simulink model "hx_model_alsop_PID"  (R2017b)
settings: Solver=FixedStepAuto  StartTime=0.0  StopTime=Tsim  FixedStep=ST  RelTol=1e-3
values from neighbouring files (symbols this model uses):
  a1 = N_stages/(3600*Mc)    (= 0.000138888888889)    [main_open_loop_step_responses.m]    (also in main_pida_vs_pid_Fp_dist.m; main_pida_vs_pid_Tci_dist.m; main_pida_vs_pid_Tpi_dist.m; main_pida_vs_pid_sp.m)
  a2 = (U*A)/(3600*Mc*Cpc)    (= 0.010660331384)    [main_open_loop_step_responses.m]    (also in main_pida_vs_pid_Fp_dist.m; main_pida_vs_pid_Tci_dist.m; main_pida_vs_pid_Tpi_dist.m; main_pida_vs_pid_sp.m)
  a3 = N_stages/(3600*Mp)    (= 0.00037037037037)    [main_open_loop_step_responses.m]    (also in main_pida_vs_pid_Fp_dist.m; main_pida_vs_pid_Tci_dist.m; main_pida_vs_pid_Tpi_dist.m; main_pida_vs_pid_sp.m)
  a4 = (U*A)/(3600*Mp*Cpp)    (= 0.0341130604288)    [main_open_loop_step_responses.m]    (also in main_pida_vs_pid_Fp_dist.m; main_pida_vs_pid_Tci_dist.m; main_pida_vs_pid_Tpi_dist.m; main_pida_vs_pid_sp.m)
  Fc = 2500/7936.64    (= 0.314994758487)    [main_open_loop_step_responses.m]    (also in main_pida_vs_pid_Fp_dist.m; main_pida_vs_pid_Tci_dist.m; main_pida_vs_pid_Tpi_dist.m; main_pida_vs_pid_sp.m)
  Fc_min = 500/7936.64    (= 0.0629989516974)    [main_open_loop_step_responses.m]    (also in main_pida_vs_pid_Fp_dist.m; main_pida_vs_pid_Tci_dist.m; main_pida_vs_pid_Tpi_dist.m; main_pida_vs_pid_sp.m)
  Fp = 1500/7936.64    (= 0.188996855092)    [main_open_loop_step_responses.m]    (also in main_pida_vs_pid_Fp_dist.m; main_pida_vs_pid_Tci_dist.m; main_pida_vs_pid_Tpi_dist.m; main_pida_vs_pid_sp.m)
  Kp = KpPID    [main_pida_vs_pid_Fp_dist.m]    (also in main_pida_vs_pid_Tci_dist.m; main_pida_vs_pid_Tpi_dist.m; main_pida_vs_pid_sp.m)
  N = 10    [main_pida_vs_pid_Fp_dist.m]    (also in main_pida_vs_pid_Tci_dist.m; main_pida_vs_pid_Tpi_dist.m; main_pida_vs_pid_sp.m; main_tuning_pid.m = 20)
  noise_max = 0.5    [main_pida_vs_pid_Fp_dist.m]    (also in main_pida_vs_pid_Tci_dist.m; main_pida_vs_pid_Tpi_dist.m; main_pida_vs_pid_sp.m)
  noise_min = -0.5    [main_pida_vs_pid_Fp_dist.m]    (also in main_pida_vs_pid_Tci_dist.m; main_pida_vs_pid_Tpi_dist.m; main_pida_vs_pid_sp.m)
  step_Fp = 0    [main_open_loop_step_responses.m]    (also in main_pida_vs_pid_Fp_dist.m = 0.0125; main_pida_vs_pid_Tci_dist.m; main_pida_vs_pid_Tpi_dist.m; main_pida_vs_pid_sp.m)
  step_Tci = 0    [main_open_loop_step_responses.m]    (also in main_pida_vs_pid_Fp_dist.m; main_pida_vs_pid_Tci_dist.m = 2.5; main_pida_vs_pid_Tpi_dist.m; main_pida_vs_pid_sp.m)
  step_time = 0    [main_open_loop_step_responses.m]    (also in main_pida_vs_pid_Fp_dist.m; main_pida_vs_pid_Tci_dist.m; main_pida_vs_pid_Tpi_dist.m; main_pida_vs_pid_sp.m)
  step_Tpi = 0    [main_open_loop_step_responses.m]    (also in main_pida_vs_pid_Fp_dist.m; main_pida_vs_pid_Tci_dist.m; main_pida_vs_pid_Tpi_dist.m = 2.5; main_pida_vs_pid_sp.m)
  step_Tpo = 0    [main_open_loop_step_responses.m]    (also in main_pida_vs_pid_Fp_dist.m; main_pida_vs_pid_Tci_dist.m; main_pida_vs_pid_Tpi_dist.m; main_pida_vs_pid_sp.m = -2.5)
  Tci = 294.26    [main_open_loop_step_responses.m]    (also in main_pida_vs_pid_Fp_dist.m; main_pida_vs_pid_Tci_dist.m; main_pida_vs_pid_Tpi_dist.m; main_pida_vs_pid_sp.m)
  Tco_init1 = Tco_init1.Data(end)    [main_open_loop_step_responses.m]    (also in main_pida_vs_pid_Fp_dist.m; main_pida_vs_pid_Tci_dist.m; main_pida_vs_pid_Tpi_dist.m; main_pida_vs_pid_sp.m)
  Tco_init10 = Tco_init10.Data(end)    [main_open_loop_step_responses.m]    (also in main_pida_vs_pid_Fp_dist.m; main_pida_vs_pid_Tci_dist.m; main_pida_vs_pid_Tpi_dist.m; main_pida_vs_pid_sp.m)
  Tco_init11 = Tco_init11.Data(end)    [main_open_loop_step_responses.m]    (also in main_pida_vs_pid_Fp_dist.m; main_pida_vs_pid_Tci_dist.m; main_pida_vs_pid_Tpi_dist.m; main_pida_vs_pid_sp.m)
  Tco_init12 = Tco_init12.Data(end)    [main_open_loop_step_responses.m]    (also in main_pida_vs_pid_Fp_dist.m; main_pida_vs_pid_Tci_dist.m; main_pida_vs_pid_Tpi_dist.m; main_pida_vs_pid_sp.m)
  Tco_init13 = Tco_init13.Data(end)    [main_open_loop_step_responses.m]    (also in main_pida_vs_pid_Fp_dist.m; main_pida_vs_pid_Tci_dist.m; main_pida_vs_pid_Tpi_dist.m; main_pida_vs_pid_sp.m)
  Tco_init14 = Tco_init14.Data(end)    [main_open_loop_step_responses.m]    (also in main_pida_vs_pid_Fp_dist.m; main_pida_vs_pid_Tci_dist.m; main_pida_vs_pid_Tpi_dist.m; main_pida_vs_pid_sp.m)
  Tco_init15 = Tco_init15.Data(end)    [main_open_loop_step_responses.m]    (also in main_pida_vs_pid_Fp_dist.m; main_pida_vs_pid_Tci_dist.m; main_pida_vs_pid_Tpi_dist.m; main_pida_vs_pid_sp.m)
  Tco_init16 = Tco_init16.Data(end)    [main_open_loop_step_responses.m]    (also in main_pida_vs_pid_Fp_dist.m; main_pida_vs_pid_Tci_dist.m; main_pida_vs_pid_Tpi_dist.m; main_pida_vs_pid_sp.m)
  Tco_init17 = Tco_init17.Data(end)    [main_open_loop_step_responses.m]    (also in main_pida_vs_pid_Fp_dist.m; main_pida_vs_pid_Tci_dist.m; main_pida_vs_pid_Tpi_dist.m; main_pida_vs_pid_sp.m)
  Tco_init18 = Tco_init18.Data(end)    [main_open_loop_step_responses.m]    (also in main_pida_vs_pid_Fp_dist.m; main_pida_vs_pid_Tci_dist.m; main_pida_vs_pid_Tpi_dist.m; main_pida_vs_pid_sp.m)
  Tco_init19 = Tco_init19.Data(end)    [main_open_loop_step_responses.m]    (also in main_pida_vs_pid_Fp_dist.m; main_pida_vs_pid_Tci_dist.m; main_pida_vs_pid_Tpi_dist.m; main_pida_vs_pid_sp.m)
  Tco_init2 = Tco_init2.Data(end)    [main_open_loop_step_responses.m]    (also in main_pida_vs_pid_Fp_dist.m; main_pida_vs_pid_Tci_dist.m; main_pida_vs_pid_Tpi_dist.m; main_pida_vs_pid_sp.m)
  Tco_init20 = Tco_init20.Data(end)    [main_open_loop_step_responses.m]    (also in main_pida_vs_pid_Fp_dist.m; main_pida_vs_pid_Tci_dist.m; main_pida_vs_pid_Tpi_dist.m; main_pida_vs_pid_sp.m)
  Tco_init3 = Tco_init3.Data(end)    [main_open_loop_step_responses.m]    (also in main_pida_vs_pid_Fp_dist.m; main_pida_vs_pid_Tci_dist.m; main_pida_vs_pid_Tpi_dist.m; main_pida_vs_pid_sp.m)
  Tco_init4 = Tco_init4.Data(end)    [main_open_loop_step_responses.m]    (also in main_pida_vs_pid_Fp_dist.m; main_pida_vs_pid_Tci_dist.m; main_pida_vs_pid_Tpi_dist.m; main_pida_vs_pid_sp.m)
  Tco_init5 = Tco_init5.Data(end)    [main_open_loop_step_responses.m]    (also in main_pida_vs_pid_Fp_dist.m; main_pida_vs_pid_Tci_dist.m; main_pida_vs_pid_Tpi_dist.m; main_pida_vs_pid_sp.m)
  Tco_init6 = Tco_init6.Data(end)    [main_open_loop_step_responses.m]    (also in main_pida_vs_pid_Fp_dist.m; main_pida_vs_pid_Tci_dist.m; main_pida_vs_pid_Tpi_dist.m; main_pida_vs_pid_sp.m)
  Tco_init7 = Tco_init7.Data(end)    [main_open_loop_step_responses.m]    (also in main_pida_vs_pid_Fp_dist.m; main_pida_vs_pid_Tci_dist.m; main_pida_vs_pid_Tpi_dist.m; main_pida_vs_pid_sp.m)
  Tco_init8 = Tco_init8.Data(end)    [main_open_loop_step_responses.m]    (also in main_pida_vs_pid_Fp_dist.m; main_pida_vs_pid_Tci_dist.m; main_pida_vs_pid_Tpi_dist.m; main_pida_vs_pid_sp.m)
  Tco_init9 = Tco_init9.Data(end)    [main_open_loop_step_responses.m]    (also in main_pida_vs_pid_Fp_dist.m; main_pida_vs_pid_Tci_dist.m; main_pida_vs_pid_Tpi_dist.m; main_pida_vs_pid_sp.m)
  Td = TdPID    [main_pida_vs_pid_Fp_dist.m]    (also in main_pida_vs_pid_Tci_dist.m; main_pida_vs_pid_Tpi_dist.m; main_pida_vs_pid_sp.m)
  Ti = TiPID    [main_pida_vs_pid_Fp_dist.m]    (also in main_pida_vs_pid_Tci_dist.m; main_pida_vs_pid_Tpi_dist.m; main_pida_vs_pid_sp.m)
  Tpi = 366.48    [main_open_loop_step_responses.m]    (also in main_pida_vs_pid_Fp_dist.m; main_pida_vs_pid_Tci_dist.m; main_pida_vs_pid_Tpi_dist.m; main_pida_vs_pid_sp.m)
  Tpo_init = (Tpo_init1 - 32)*(5/9) + 273.15    [main_open_loop_step_responses.m]    (also in main_pida_vs_pid_Fp_dist.m; main_pida_vs_pid_Tci_dist.m; main_pida_vs_pid_Tpi_dist.m; main_pida_vs_pid_sp.m)
  Tpo_init1 = Tpo_init1.Data(end)    [main_open_loop_step_responses.m]    (also in main_pida_vs_pid_Fp_dist.m; main_pida_vs_pid_Tci_dist.m; main_pida_vs_pid_Tpi_dist.m; main_pida_vs_pid_sp.m)
  Tpo_init10 = Tpo_init10.Data(end)    [main_open_loop_step_responses.m]    (also in main_pida_vs_pid_Fp_dist.m; main_pida_vs_pid_Tci_dist.m; main_pida_vs_pid_Tpi_dist.m; main_pida_vs_pid_sp.m)
  Tpo_init11 = Tpo_init11.Data(end)    [main_open_loop_step_responses.m]    (also in main_pida_vs_pid_Fp_dist.m; main_pida_vs_pid_Tci_dist.m; main_pida_vs_pid_Tpi_dist.m; main_pida_vs_pid_sp.m)
  Tpo_init12 = Tpo_init12.Data(end)    [main_open_loop_step_responses.m]    (also in main_pida_vs_pid_Fp_dist.m; main_pida_vs_pid_Tci_dist.m; main_pida_vs_pid_Tpi_dist.m; main_pida_vs_pid_sp.m)
  Tpo_init13 = Tpo_init13.Data(end)    [main_open_loop_step_responses.m]    (also in main_pida_vs_pid_Fp_dist.m; main_pida_vs_pid_Tci_dist.m; main_pida_vs_pid_Tpi_dist.m; main_pida_vs_pid_sp.m)
  Tpo_init14 = Tpo_init14.Data(end)    [main_open_loop_step_responses.m]    (also in main_pida_vs_pid_Fp_dist.m; main_pida_vs_pid_Tci_dist.m; main_pida_vs_pid_Tpi_dist.m; main_pida_vs_pid_sp.m)
  Tpo_init15 = Tpo_init15.Data(end)    [main_open_loop_step_responses.m]    (also in main_pida_vs_pid_Fp_dist.m; main_pida_vs_pid_Tci_dist.m; main_pida_vs_pid_Tpi_dist.m; main_pida_vs_pid_sp.m)
  Tpo_init16 = Tpo_init16.Data(end)    [main_open_loop_step_responses.m]    (also in main_pida_vs_pid_Fp_dist.m; main_pida_vs_pid_Tci_dist.m; main_pida_vs_pid_Tpi_dist.m; main_pida_vs_pid_sp.m)
  Tpo_init17 = Tpo_init17.Data(end)    [main_open_loop_step_responses.m]    (also in main_pida_vs_pid_Fp_dist.m; main_pida_vs_pid_Tci_dist.m; main_pida_vs_pid_Tpi_dist.m; main_pida_vs_pid_sp.m)
  Tpo_init18 = Tpo_init18.Data(end)    [main_open_loop_step_responses.m]    (also in main_pida_vs_pid_Fp_dist.m; main_pida_vs_pid_Tci_dist.m; main_pida_vs_pid_Tpi_dist.m; main_pida_vs_pid_sp.m)
  Tpo_init19 = Tpo_init19.Data(end)    [main_open_loop_step_responses.m]    (also in main_pida_vs_pid_Fp_dist.m; main_pida_vs_pid_Tci_dist.m; main_pida_vs_pid_Tpi_dist.m; main_pida_vs_pid_sp.m)
  Tpo_init2 = Tpo_init2.Data(end)    [main_open_loop_step_responses.m]    (also in main_pida_vs_pid_Fp_dist.m; main_pida_vs_pid_Tci_dist.m; main_pida_vs_pid_Tpi_dist.m; main_pida_vs_pid_sp.m)
  Tpo_init20 = Tpo_init20.Data(end)    [main_open_loop_step_responses.m]    (also in main_pida_vs_pid_Fp_dist.m; main_pida_vs_pid_Tci_dist.m; main_pida_vs_pid_Tpi_dist.m; main_pida_vs_pid_sp.m)
  Tpo_init3 = Tpo_init3.Data(end)    [main_open_loop_step_responses.m]    (also in main_pida_vs_pid_Fp_dist.m; main_pida_vs_pid_Tci_dist.m; main_pida_vs_pid_Tpi_dist.m; main_pida_vs_pid_sp.m)
  Tpo_init4 = Tpo_init4.Data(end)    [main_open_loop_step_responses.m]    (also in main_pida_vs_pid_Fp_dist.m; main_pida_vs_pid_Tci_dist.m; main_pida_vs_pid_Tpi_dist.m; main_pida_vs_pid_sp.m)
  Tpo_init5 = Tpo_init5.Data(end)    [main_open_loop_step_responses.m]    (also in main_pida_vs_pid_Fp_dist.m; main_pida_vs_pid_Tci_dist.m; main_pida_vs_pid_Tpi_dist.m; main_pida_vs_pid_sp.m)
  Tpo_init6 = Tpo_init6.Data(end)    [main_open_loop_step_responses.m]    (also in main_pida_vs_pid_Fp_dist.m; main_pida_vs_pid_Tci_dist.m; main_pida_vs_pid_Tpi_dist.m; main_pida_vs_pid_sp.m)
  Tpo_init7 = Tpo_init7.Data(end)    [main_open_loop_step_responses.m]    (also in main_pida_vs_pid_Fp_dist.m; main_pida_vs_pid_Tci_dist.m; main_pida_vs_pid_Tpi_dist.m; main_pida_vs_pid_sp.m)
  Tpo_init8 = Tpo_init8.Data(end)    [main_open_loop_step_responses.m]    (also in main_pida_vs_pid_Fp_dist.m; main_pida_vs_pid_Tci_dist.m; main_pida_vs_pid_Tpi_dist.m; main_pida_vs_pid_sp.m)
  Tpo_init9 = Tpo_init9.Data(end)    [main_open_loop_step_responses.m]    (also in main_pida_vs_pid_Fp_dist.m; main_pida_vs_pid_Tci_dist.m; main_pida_vs_pid_Tpi_dist.m; main_pida_vs_pid_sp.m)
  Wgc = WcpPID    [main_pida_vs_pid_Fp_dist.m]    (also in main_pida_vs_pid_Tci_dist.m; main_pida_vs_pid_Tpi_dist.m; main_pida_vs_pid_sp.m)
  x_eq = -(A_f\(B_f*Fc))    [main_pida_vs_pid_Fp_dist.m]    (also in main_pida_vs_pid_Tci_dist.m; main_pida_vs_pid_Tpi_dist.m; main_pida_vs_pid_sp.m)
undefined symbols (not defined in the file or in its folder): A_f, B_f, C_f, D_f
(part 1 of 2)
settings Model: Creator=Michele  LastModifiedBy=Michele

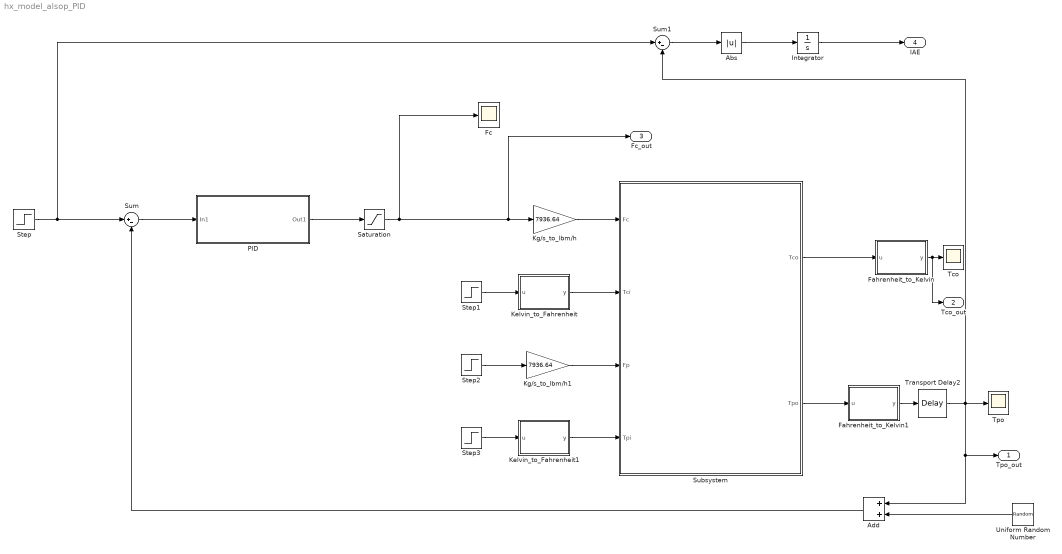
== system hx_model_alsop_PID ==
  Abs : Abs
  Add : Sum
  Fahrenheit_to_Kelvin : MATLAB Function  TreatAsAtomicUnit=on
  Fahrenheit_to_Kelvin1 : MATLAB Function  TreatAsAtomicUnit=on
  Fc : Scope
  Integrator : Integrator
  Kelvin_to_Fahrenheit : MATLAB Function  TreatAsAtomicUnit=on
  Kelvin_to_Fahrenheit1 : MATLAB Function  TreatAsAtomicUnit=on
  Kg/s_to_lbm/h : Gain  Gain=7936.64
  Kg/s_to_lbm/h1 : Gain  Gain=7936.64
  PID : Subsystem
  Saturation : Saturate  UpperLimit=inf  LowerLimit=Fc_min
  Step : Step  Time=step_time  Before=Tpo_init  After=Tpo_init+step_Tpo  SampleTime=0
  Step1 : Step  Time=step_time  Before=Tci  After=Tci+step_Tci  SampleTime=0
  Step2 : Step  Time=step_time  Before=Fp  After=Fp+step_Fp  SampleTime=0
  Step3 : Step  Time=step_time  Before=Tpi  After=Tpi+step_Tpi  SampleTime=0
  Subsystem : Subsystem
  Sum : Sum  Inputs=|+-
  Sum1 : Sum  Inputs=|+-
  Tco : Scope
  Tpo : Scope
  Transport Delay2 : TransportDelay  DelayTime=35  InitialOutput=(Tpo_init1 - 32)*(5/9) + 273.15
  Uniform Random Number : UniformRandomNumber  Minimum=noise_min  Maximum=noise_max  SampleTime=0.1
  Tpo_out : Outport
  Tco_out : Outport  Port=2
  Fc_out : Outport  Port=3
  IAE : Outport  Port=4
  wires:
  Step2/1 -> Kg/s_to_lbm/h1/1
  Step3/1 -> Kelvin_to_Fahrenheit1/1(u)
  Step1/1 -> Kelvin_to_Fahrenheit/1(u)
  Kelvin_to_Fahrenheit/1(y) -> Subsystem/2(Tci)
  Kelvin_to_Fahrenheit1/1(y) -> Subsystem/4(Tpi)
  Fahrenheit_to_Kelvin/1(y) -> Tco_out/1, Tco/1
  Fahrenheit_to_Kelvin1/1(y) -> Transport Delay2/1
  Kg/s_to_lbm/h/1 -> Subsystem/1(Fc)
  Kg/s_to_lbm/h1/1 -> Subsystem/3(Fp)
  Subsystem/1(Tco) -> Fahrenheit_to_Kelvin/1(u)
  Subsystem/2(Tpo) -> Fahrenheit_to_Kelvin1/1(u)
  Saturation/1 -> Fc_out/1, Kg/s_to_lbm/h/1, Fc/1
  PID/1(Out1) -> Saturation/1
  Step/1 -> Sum1/1, Sum/1
  Abs/1 -> Integrator/1
  Sum/1 -> PID/1(In1)
  Integrator/1 -> IAE/1
  Add/1 -> Sum/2
  Uniform Random Number/1 -> Add/2
  Sum1/1 -> Abs/1
  Transport Delay2/1 -> Sum1/2, Tpo/1, Tpo_out/1, Add/1

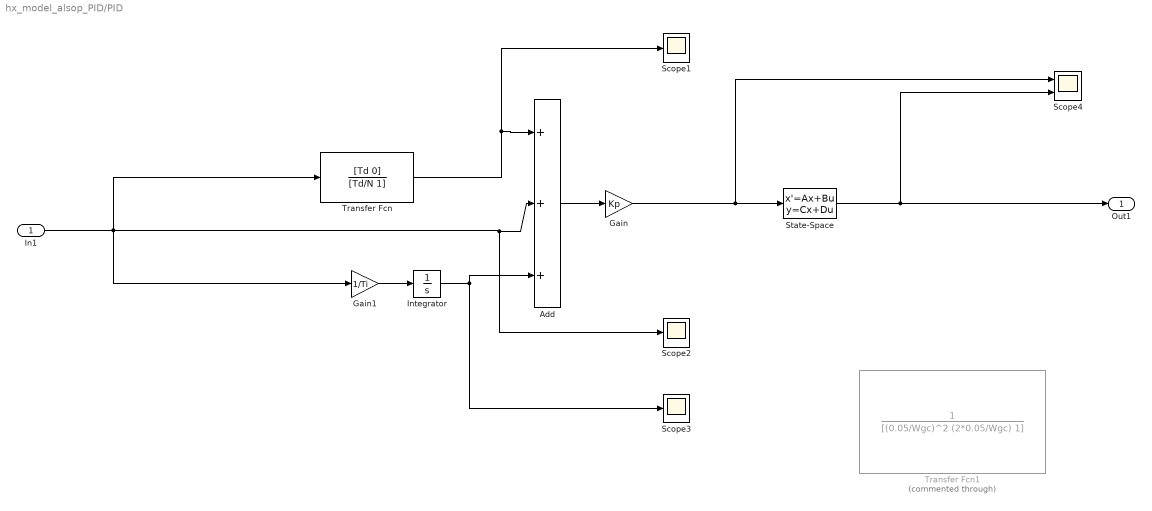
== system hx_model_alsop_PID/PID ==
  In1 : Inport
  Add : Sum  Inputs=+++
  Gain : Gain  Gain=Kp
  Gain1 : Gain  Gain=1/Ti
  Integrator : Integrator  InitialCondition=Fc/Kp
  Scope1 : Scope
  Scope2 : Scope
  Scope3 : Scope
  Scope4 : Scope  NumInputPorts=2
  State-Space : StateSpace  A=A_f  B=B_f  C=C_f  D=D_f  InitialCondition=x_eq
  Transfer Fcn : TransferFcn  Numerator=[Td 0]  Denominator=[Td/N 1]
  Transfer Fcn1 : TransferFcn  Commented=through  Denominator=[(0.05/Wgc)^2 (2*0.05/Wgc) 1]
  Out1 : Outport
  wires:
  Add/1 -> Gain/1
  Integrator/1 -> Add/3, Scope3/1
  Gain1/1 -> Integrator/1
  State-Space/1 -> Scope4/2, Out1/1
  In1/1 -> Transfer Fcn/1, Gain1/1, Add/2, Scope2/1
  Transfer Fcn/1 -> Add/1, Scope1/1
  Gain/1 -> Scope4/1, State-Space/1

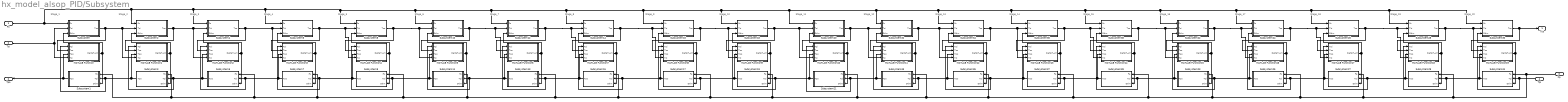
== system hx_model_alsop_PID/Subsystem ==
  note: Stage_1
  note: Stage_2
  note: Stage_3
  note: Stage_4
  note: Stage_5
  note: Stage_6
  note: Stage_7
  note: Stage_8
  note: Stage_9
  note: Stage_10
  note: Stage_13
  note: Stage_20
  note: Stage_16
  note: Stage_11
  note: Stage_18
  note: Stage_15
  note: Stage_19
  note: Stage_12
  note: Stage_17
  note: Stage_14
  Fc : Inport
  Tci : Inport  Port=2
  Fp : Inport  Port=3
  Tpi : Inport  Port=4
  MATLAB Function : MATLAB Function  TreatAsAtomicUnit=on
  MATLAB Function1 : MATLAB Function  TreatAsAtomicUnit=on
  MATLAB Function10 : MATLAB Function  TreatAsAtomicUnit=on
  MATLAB Function11 : MATLAB Function  TreatAsAtomicUnit=on
  MATLAB Function12 : MATLAB Function  TreatAsAtomicUnit=on
  MATLAB Function13 : MATLAB Function  TreatAsAtomicUnit=on
  MATLAB Function14 : MATLAB Function  TreatAsAtomicUnit=on
  MATLAB Function15 : MATLAB Function  TreatAsAtomicUnit=on
  MATLAB Function16 : MATLAB Function  TreatAsAtomicUnit=on
  MATLAB Function17 : MATLAB Function  TreatAsAtomicUnit=on
  MATLAB Function18 : MATLAB Function  TreatAsAtomicUnit=on
  MATLAB Function19 : MATLAB Function  TreatAsAtomicUnit=on
  MATLAB Function2 : MATLAB Function  TreatAsAtomicUnit=on
  MATLAB Function3 : MATLAB Function  TreatAsAtomicUnit=on
  MATLAB Function4 : MATLAB Function  TreatAsAtomicUnit=on
  MATLAB Function5 : MATLAB Function  TreatAsAtomicUnit=on
  MATLAB Function6 : MATLAB Function  TreatAsAtomicUnit=on
  MATLAB Function7 : MATLAB Function  TreatAsAtomicUnit=on
  MATLAB Function8 : MATLAB Function  TreatAsAtomicUnit=on
  MATLAB Function9 : MATLAB Function  TreatAsAtomicUnit=on
  Subsystem : Subsystem
  Subsystem1 : Subsystem
  Subsystem10 : Subsystem
  Subsystem11 : Subsystem
  Subsystem12 : Subsystem
  Subsystem13 : Subsystem
  Subsystem14 : Subsystem
  Subsystem15 : Subsystem
  Subsystem16 : Subsystem
  Subsystem17 : Subsystem
  Subsystem18 : Subsystem
  Subsystem19 : Subsystem
  Subsystem2 : Subsystem
  Subsystem20 : Subsystem
  Subsystem21 : Subsystem
  Subsystem22 : Subsystem
  Subsystem23 : Subsystem
  Subsystem24 : Subsystem
  Subsystem25 : Subsystem
  Subsystem26 : Subsystem
  Subsystem27 : Subsystem
  Subsystem28 : Subsystem
  Subsystem29 : Subsystem
  Subsystem3 : Subsystem
  Subsystem30 : Subsystem
  Subsystem31 : Subsystem
  Subsystem32 : Subsystem
  Subsystem33 : Subsystem
  Subsystem34 : Subsystem
  Subsystem35 : Subsystem
  Subsystem36 : Subsystem
  Subsystem37 : Subsystem
  Subsystem38 : Subsystem
  Subsystem39 : Subsystem
  Subsystem4 : Subsystem
  Subsystem5 : Subsystem
  Subsystem6 : Subsystem
  Subsystem7 : Subsystem
  Subsystem8 : Subsystem
  Subsystem9 : Subsystem
  Tco : Outport
  Tpo : Outport  Port=2
  wires:
  Subsystem1/1(Tpo) -> Tpo/1, MATLAB Function/3(Tpo)
  Subsystem/1(Tco) -> MATLAB Function/2(Tco), MATLAB Function1/4(Tci), Subsystem2/2(Tci)
  MATLAB Function/1(DeltaT_LM) -> Subsystem1/3(Dtlm), Subsystem/3(Dtlm)
  Tci/1 -> MATLAB Function/4(Tci), Subsystem/2(Tci)
  MATLAB Function1/1(DeltaT_LM) -> Subsystem2/3(Dtlm), Subsystem3/3(Dtlm)
  Subsystem2/1(Tco) -> MATLAB Function2/4(Tci), Subsystem4/2(Tci), MATLAB Function1/2(Tco)
  Subsystem3/1(Tpo) -> MATLAB Function/1(Tpi), Subsystem1/2(Tpi), MATLAB Function1/3(Tpo)
  Subsystem4/1(Tco) -> MATLAB Function2/2(Tco), MATLAB Function3/4(Tci), Subsystem6/2(Tci)
  MATLAB Function2/1(DeltaT_LM) -> Subsystem5/3(Dtlm), Subsystem4/3(Dtlm)
  MATLAB Function3/1(DeltaT_LM) -> Subsystem6/3(Dtlm), Subsystem7/3(Dtlm)
  Subsystem6/1(Tco) -> MATLAB Function4/4(Tci), Subsystem8/2(Tci), MATLAB Function3/2(Tco)
  Subsystem8/1(Tco) -> MATLAB Function5/4(Tci), Subsystem10/2(Tci), MATLAB Function4/2(Tco)
  MATLAB Function4/1(DeltaT_LM) -> Subsystem9/3(Dtlm), Subsystem8/3(Dtlm)
  MATLAB Function5/1(DeltaT_LM) -> Subsystem10/3(Dtlm), Subsystem11/3(Dtlm)
  Subsystem10/1(Tco) -> MATLAB Function6/4(Tci), Subsystem12/2(Tci), MATLAB Function5/2(Tco)
  Subsystem12/1(Tco) -> MATLAB Function7/4(Tci), Subsystem14/2(Tci), MATLAB Function6/2(Tco)
  MATLAB Function6/1(DeltaT_LM) -> Subsystem13/3(Dtlm), Subsystem12/3(Dtlm)
  MATLAB Function7/1(DeltaT_LM) -> Subsystem14/3(Dtlm), Subsystem15/3(Dtlm)
  Subsystem14/1(Tco) -> MATLAB Function8/4(Tci), Subsystem16/2(Tci), MATLAB Function7/2(Tco)
  Subsystem16/1(Tco) -> MATLAB Function9/4(Tci), Subsystem18/2(Tci), MATLAB Function8/2(Tco)
  MATLAB Function8/1(DeltaT_LM) -> Subsystem17/3(Dtlm), Subsystem16/3(Dtlm)
  MATLAB Function9/1(DeltaT_LM) -> Subsystem18/3(Dtlm), Subsystem19/3(Dtlm)
  Subsystem5/1(Tpo) -> MATLAB Function2/3(Tpo), MATLAB Function1/1(Tpi), Subsystem3/2(Tpi)
  Subsystem7/1(Tpo) -> MATLAB Function2/1(Tpi), Subsystem5/2(Tpi), MATLAB Function3/3(Tpo)
  Subsystem9/1(Tpo) -> MATLAB Function3/1(Tpi), Subsystem7/2(Tpi), MATLAB Function4/3(Tpo)
  Subsystem11/1(Tpo) -> MATLAB Function4/1(Tpi), Subsystem9/2(Tpi), MATLAB Function5/3(Tpo)
  Subsystem13/1(Tpo) -> MATLAB Function5/1(Tpi), Subsystem11/2(Tpi), MATLAB Function6/3(Tpo)
  Subsystem15/1(Tpo) -> MATLAB Function6/1(Tpi), Subsystem13/2(Tpi), MATLAB Function7/3(Tpo)
  Subsystem17/1(Tpo) -> MATLAB Function7/1(Tpi), Subsystem15/2(Tpi), MATLAB Function8/3(Tpo)
  Subsystem19/1(Tpo) -> MATLAB Function8/1(Tpi), Subsystem17/2(Tpi), MATLAB Function9/3(Tpo)
  Subsystem31/1(Tpo) -> MATLAB Function18/1(Tpi), Subsystem29/2(Tpi), MATLAB Function19/3(Tpo)
  Subsystem32/1(Tco) -> MATLAB Function12/4(Tci), Subsystem34/2(Tci), MATLAB Function11/2(Tco)
  MATLAB Function11/1(DeltaT_LM) -> Subsystem32/3(Dtlm), Subsystem33/3(Dtlm)
  Subsystem25/1(Tpo) -> MATLAB Function15/1(Tpi), Subsystem23/2(Tpi), MATLAB Function16/3(Tpo)
  MATLAB Function15/1(DeltaT_LM) -> Subsystem22/3(Dtlm), Subsystem23/3(Dtlm)
  MATLAB Function12/1(DeltaT_LM) -> Subsystem35/3(Dtlm), Subsystem34/3(Dtlm)
  Subsystem33/1(Tpo) -> MATLAB Function10/1(Tpi), Subsystem21/2(Tpi), MATLAB Function11/3(Tpo)
  MATLAB Function14/1(DeltaT_LM) -> Subsystem39/3(Dtlm), Subsystem38/3(Dtlm)
  Subsystem34/1(Tco) -> MATLAB Function12/2(Tco), MATLAB Function13/4(Tci), Subsystem36/2(Tci)
  Fc/1 -> Subsystem30/1(Fc), Subsystem28/1(Fc), Subsystem26/1(Fc), Subsystem24/1(Fc), Subsystem22/1(Fc), Subsystem38/1(Fc), Subsystem36/1(Fc), Subsystem34/1(Fc), Subsystem32/1(Fc), Subsystem20/1(Fc), Subsystem18/1(Fc), Subsystem16/1(Fc), Subsystem14/1(Fc), Subsystem12/1(Fc), Subsystem10/1(Fc), Subsystem8/1(Fc), Subsystem6/1(Fc), Subsystem4/1(Fc), Subsystem2/1(Fc), Subsystem/1(Fc)
  Subsystem18/1(Tco) -> MATLAB Function9/2(Tco), MATLAB Function10/4(Tci), Subsystem20/2(Tci)
  Subsystem20/1(Tco) -> MATLAB Function10/2(Tco), MATLAB Function11/4(Tci), Subsystem32/2(Tci)
  MATLAB Function10/1(DeltaT_LM) -> Subsystem21/3(Dtlm), Subsystem20/3(Dtlm)
  Subsystem23/1(Tpo) -> MATLAB Function14/1(Tpi), Subsystem39/2(Tpi), MATLAB Function15/3(Tpo)
  Subsystem37/1(Tpo) -> MATLAB Function12/1(Tpi), Subsystem35/2(Tpi), MATLAB Function13/3(Tpo)
  Subsystem38/1(Tco) -> MATLAB Function15/4(Tci), Subsystem22/2(Tci), MATLAB Function14/2(Tco)
  Subsystem21/1(Tpo) -> MATLAB Function10/3(Tpo), MATLAB Function9/1(Tpi), Subsystem19/2(Tpi)
  Subsystem29/1(Tpo) -> MATLAB Function17/1(Tpi), Subsystem27/2(Tpi), MATLAB Function18/3(Tpo)
  Subsystem27/1(Tpo) -> MATLAB Function16/1(Tpi), Subsystem25/2(Tpi), MATLAB Function17/3(Tpo)
  Subsystem22/1(Tco) -> MATLAB Function16/4(Tci), Subsystem24/2(Tci), MATLAB Function15/2(Tco)
  MATLAB Function16/1(DeltaT_LM) -> Subsystem25/3(Dtlm), Subsystem24/3(Dtlm)
  MATLAB Function17/1(DeltaT_LM) -> Subsystem26/3(Dtlm), Subsystem27/3(Dtlm)
  Subsystem24/1(Tco) -> MATLAB Function17/4(Tci), Subsystem26/2(Tci), MATLAB Function16/2(Tco)
  Subsystem30/1(Tco) -> MATLAB Function19/2(Tco), Tco/1
  Subsystem35/1(Tpo) -> MATLAB Function12/3(Tpo), MATLAB Function11/1(Tpi), Subsystem33/2(Tpi)
  Subsystem39/1(Tpo) -> MATLAB Function13/1(Tpi), Subsystem37/2(Tpi), MATLAB Function14/3(Tpo)
  Subsystem26/1(Tco) -> MATLAB Function18/4(Tci), Subsystem28/2(Tci), MATLAB Function17/2(Tco)
  MATLAB Function19/1(DeltaT_LM) -> Subsystem30/3(Dtlm), Subsystem31/3(Dtlm)
  MATLAB Function13/1(DeltaT_LM) -> Subsystem36/3(Dtlm), Subsystem37/3(Dtlm)
  Subsystem36/1(Tco) -> MATLAB Function14/4(Tci), Subsystem38/2(Tci), MATLAB Function13/2(Tco)
  Subsystem28/1(Tco) -> MATLAB Function19/4(Tci), Subsystem30/2(Tci), MATLAB Function18/2(Tco)
  MATLAB Function18/1(DeltaT_LM) -> Subsystem29/3(Dtlm), Subsystem28/3(Dtlm)
  Tpi/1 -> MATLAB Function19/1(Tpi), Subsystem31/2(Tpi)
  Fp/1 -> Subsystem1/1(Fp), Subsystem3/1(Fp), Subsystem5/1(Fp), Subsystem7/1(Fp), Subsystem9/1(Fp), Subsystem11/1(Fp), Subsystem13/1(Fp), Subsystem15/1(Fp), Subsystem17/1(Fp), Subsystem19/1(Fp), Subsystem21/1(Fp), Subsystem33/1(Fp), Subsystem35/1(Fp), Subsystem37/1(Fp), Subsystem39/1(Fp), Subsystem23/1(Fp), Subsystem25/1(Fp), Subsystem27/1(Fp), Subsystem29/1(Fp), Subsystem31/1(Fp)

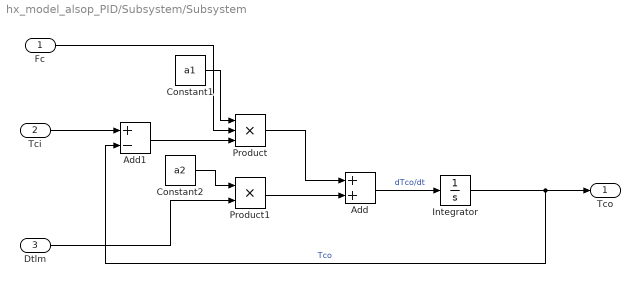
== system hx_model_alsop_PID/Subsystem/Subsystem ==
  Fc : Inport
  Tci : Inport  Port=2
  Dtlm : Inport  Port=3
  Add : Sum
  Add1 : Sum  Inputs=+-
  Constant1 : Constant  Value=a1
  Constant2 : Constant  Value=a2
  Integrator : Integrator  InitialCondition=Tco_init1
  Product : Product  Inputs=3
  Product1 : Product
  Tco : Outport
  wires:
  Dtlm/1 -> Product1/2
  Integrator/1 -> Tco/1, Add1/2  "Tco"
  Product/1 -> Add/1
  Tci/1 -> Add1/1
  Add1/1 -> Product/3
  Product1/1 -> Add/2
  Constant2/1 -> Product1/1
  Constant1/1 -> Product/1
  Add/1 -> Integrator/1  "dTco/dt"
  Fc/1 -> Product/2

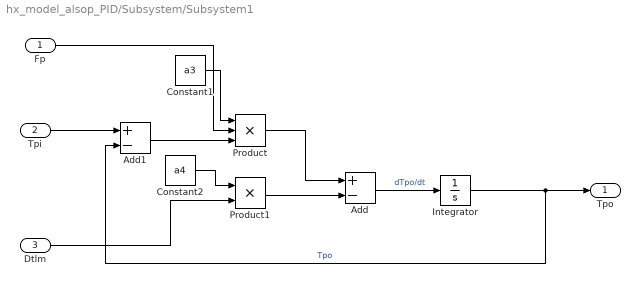
== system hx_model_alsop_PID/Subsystem/Subsystem1 ==
  Fp : Inport
  Tpi : Inport  Port=2
  Dtlm : Inport  Port=3
  Add : Sum  Inputs=+-
  Add1 : Sum  Inputs=+-
  Constant1 : Constant  Value=a3
  Constant2 : Constant  Value=a4
  Integrator : Integrator  InitialCondition=Tpo_init1
  Product : Product  Inputs=3
  Product1 : Product
  Tpo : Outport
  wires:
  Fp/1 -> Product/2
  Add/1 -> Integrator/1  "dTpo/dt"
  Constant1/1 -> Product/1
  Constant2/1 -> Product1/1
  Product1/1 -> Add/2
  Add1/1 -> Product/3
  Tpi/1 -> Add1/1
  Product/1 -> Add/1
  Integrator/1 -> Add1/2, Tpo/1  "Tpo"
  Dtlm/1 -> Product1/2

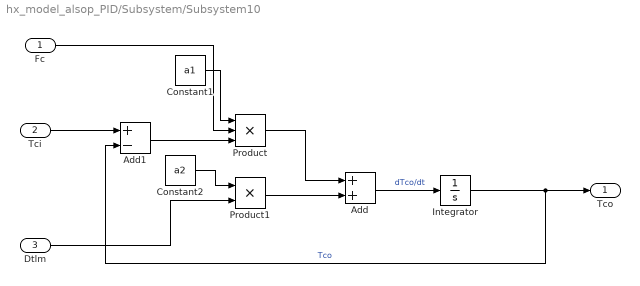
== system hx_model_alsop_PID/Subsystem/Subsystem10 ==
  Fc : Inport
  Tci : Inport  Port=2
  Dtlm : Inport  Port=3
  Add : Sum
  Add1 : Sum  Inputs=+-
  Constant1 : Constant  Value=a1
  Constant2 : Constant  Value=a2
  Integrator : Integrator  InitialCondition=Tco_init6
  Product : Product  Inputs=3
  Product1 : Product
  Tco : Outport
  wires:
  Fc/1 -> Product/2
  Add/1 -> Integrator/1  "dTco/dt"
  Constant1/1 -> Product/1
  Constant2/1 -> Product1/1
  Product1/1 -> Add/2
  Add1/1 -> Product/3
  Tci/1 -> Add1/1
  Product/1 -> Add/1
  Integrator/1 -> Add1/2, Tco/1  "Tco"
  Dtlm/1 -> Product1/2

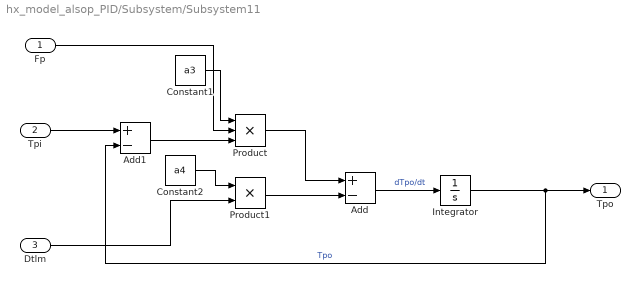
== system hx_model_alsop_PID/Subsystem/Subsystem11 ==
  Fp : Inport
  Tpi : Inport  Port=2
  Dtlm : Inport  Port=3
  Add : Sum  Inputs=+-
  Add1 : Sum  Inputs=+-
  Constant1 : Constant  Value=a3
  Constant2 : Constant  Value=a4
  Integrator : Integrator  InitialCondition=Tpo_init6
  Product : Product  Inputs=3
  Product1 : Product
  Tpo : Outport
  wires:
  Dtlm/1 -> Product1/2
  Integrator/1 -> Tpo/1, Add1/2  "Tpo"
  Product/1 -> Add/1
  Tpi/1 -> Add1/1
  Add1/1 -> Product/3
  Product1/1 -> Add/2
  Constant2/1 -> Product1/1
  Constant1/1 -> Product/1
  Add/1 -> Integrator/1  "dTpo/dt"
  Fp/1 -> Product/2

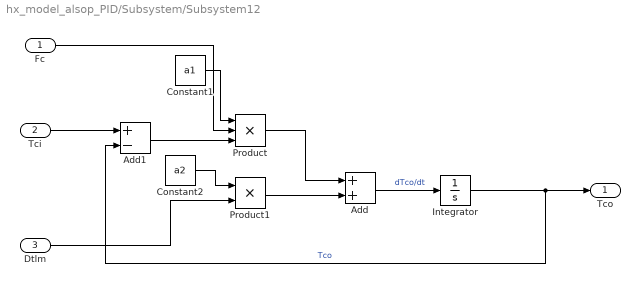
== system hx_model_alsop_PID/Subsystem/Subsystem12 ==
  Fc : Inport
  Tci : Inport  Port=2
  Dtlm : Inport  Port=3
  Add : Sum
  Add1 : Sum  Inputs=+-
  Constant1 : Constant  Value=a1
  Constant2 : Constant  Value=a2
  Integrator : Integrator  InitialCondition=Tco_init7
  Product : Product  Inputs=3
  Product1 : Product
  Tco : Outport
  wires:
  Dtlm/1 -> Product1/2
  Integrator/1 -> Tco/1, Add1/2  "Tco"
  Product/1 -> Add/1
  Tci/1 -> Add1/1
  Add1/1 -> Product/3
  Product1/1 -> Add/2
  Constant2/1 -> Product1/1
  Constant1/1 -> Product/1
  Add/1 -> Integrator/1  "dTco/dt"
  Fc/1 -> Product/2

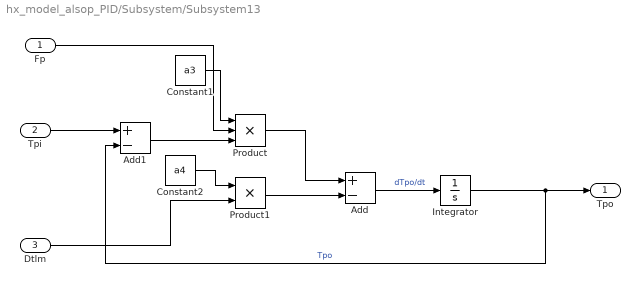
== system hx_model_alsop_PID/Subsystem/Subsystem13 ==
  Fp : Inport
  Tpi : Inport  Port=2
  Dtlm : Inport  Port=3
  Add : Sum  Inputs=+-
  Add1 : Sum  Inputs=+-
  Constant1 : Constant  Value=a3
  Constant2 : Constant  Value=a4
  Integrator : Integrator  InitialCondition=Tpo_init7
  Product : Product  Inputs=3
  Product1 : Product
  Tpo : Outport
  wires:
  Fp/1 -> Product/2
  Add/1 -> Integrator/1  "dTpo/dt"
  Constant1/1 -> Product/1
  Constant2/1 -> Product1/1
  Product1/1 -> Add/2
  Add1/1 -> Product/3
  Tpi/1 -> Add1/1
  Product/1 -> Add/1
  Integrator/1 -> Add1/2, Tpo/1  "Tpo"
  Dtlm/1 -> Product1/2

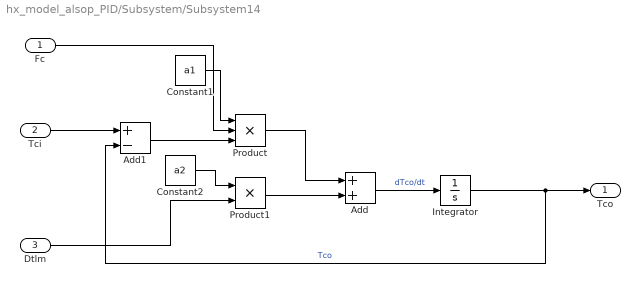
== system hx_model_alsop_PID/Subsystem/Subsystem14 ==
  Fc : Inport
  Tci : Inport  Port=2
  Dtlm : Inport  Port=3
  Add : Sum
  Add1 : Sum  Inputs=+-
  Constant1 : Constant  Value=a1
  Constant2 : Constant  Value=a2
  Integrator : Integrator  InitialCondition=Tco_init8
  Product : Product  Inputs=3
  Product1 : Product
  Tco : Outport
  wires:
  Fc/1 -> Product/2
  Add/1 -> Integrator/1  "dTco/dt"
  Constant1/1 -> Product/1
  Constant2/1 -> Product1/1
  Product1/1 -> Add/2
  Add1/1 -> Product/3
  Tci/1 -> Add1/1
  Product/1 -> Add/1
  Integrator/1 -> Add1/2, Tco/1  "Tco"
  Dtlm/1 -> Product1/2

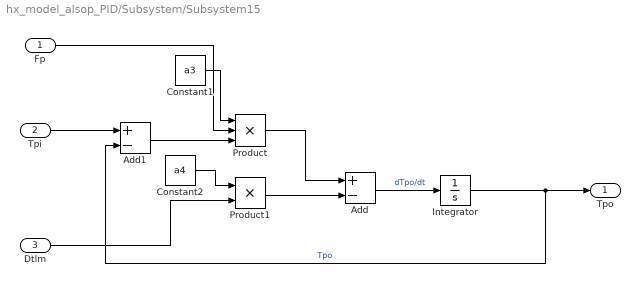
== system hx_model_alsop_PID/Subsystem/Subsystem15 ==
  Fp : Inport
  Tpi : Inport  Port=2
  Dtlm : Inport  Port=3
  Add : Sum  Inputs=+-
  Add1 : Sum  Inputs=+-
  Constant1 : Constant  Value=a3
  Constant2 : Constant  Value=a4
  Integrator : Integrator  InitialCondition=Tpo_init8
  Product : Product  Inputs=3
  Product1 : Product
  Tpo : Outport
  wires:
  Dtlm/1 -> Product1/2
  Integrator/1 -> Tpo/1, Add1/2  "Tpo"
  Product/1 -> Add/1
  Tpi/1 -> Add1/1
  Add1/1 -> Product/3
  Product1/1 -> Add/2
  Constant2/1 -> Product1/1
  Constant1/1 -> Product/1
  Add/1 -> Integrator/1  "dTpo/dt"
  Fp/1 -> Product/2

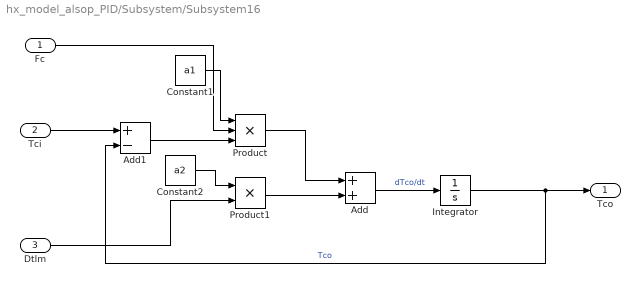
== system hx_model_alsop_PID/Subsystem/Subsystem16 ==
  Fc : Inport
  Tci : Inport  Port=2
  Dtlm : Inport  Port=3
  Add : Sum
  Add1 : Sum  Inputs=+-
  Constant1 : Constant  Value=a1
  Constant2 : Constant  Value=a2
  Integrator : Integrator  InitialCondition=Tco_init9
  Product : Product  Inputs=3
  Product1 : Product
  Tco : Outport
  wires:
  Dtlm/1 -> Product1/2
  Integrator/1 -> Tco/1, Add1/2  "Tco"
  Product/1 -> Add/1
  Tci/1 -> Add1/1
  Add1/1 -> Product/3
  Product1/1 -> Add/2
  Constant2/1 -> Product1/1
  Constant1/1 -> Product/1
  Add/1 -> Integrator/1  "dTco/dt"
  Fc/1 -> Product/2

== system hx_model_alsop_PID/Subsystem/Subsystem17 ==
  Fp : Inport
  Tpi : Inport  Port=2
  Dtlm : Inport  Port=3
  Add : Sum  Inputs=+-
  Add1 : Sum  Inputs=+-
  Constant1 : Constant  Value=a3
  Constant2 : Constant  Value=a4
  Integrator : Integrator  InitialCondition=Tpo_init9
  Product : Product  Inputs=3
  Product1 : Product
  Tpo : Outport
  wires:
  Fp/1 -> Product/2
  Add/1 -> Integrator/1  "dTpo/dt"
  Constant1/1 -> Product/1
  Constant2/1 -> Product1/1
  Product1/1 -> Add/2
  Add1/1 -> Product/3
  Tpi/1 -> Add1/1
  Product/1 -> Add/1
  Integrator/1 -> Add1/2, Tpo/1  "Tpo"
  Dtlm/1 -> Product1/2

== system hx_model_alsop_PID/Subsystem/Subsystem18 ==
  Fc : Inport
  Tci : Inport  Port=2
  Dtlm : Inport  Port=3
  Add : Sum
  Add1 : Sum  Inputs=+-
  Constant1 : Constant  Value=a1
  Constant2 : Constant  Value=a2
  Integrator : Integrator  InitialCondition=Tco_init10
  Product : Product  Inputs=3
  Product1 : Product
  Tco : Outport
  wires:
  Fc/1 -> Product/2
  Add/1 -> Integrator/1  "dTco/dt"
  Constant1/1 -> Product/1
  Constant2/1 -> Product1/1
  Product1/1 -> Add/2
  Add1/1 -> Product/3
  Tci/1 -> Add1/1
  Product/1 -> Add/1
  Integrator/1 -> Add1/2, Tco/1  "Tco"
  Dtlm/1 -> Product1/2

== system hx_model_alsop_PID/Subsystem/Subsystem19 ==
  Fp : Inport
  Tpi : Inport  Port=2
  Dtlm : Inport  Port=3
  Add : Sum  Inputs=+-
  Add1 : Sum  Inputs=+-
  Constant1 : Constant  Value=a3
  Constant2 : Constant  Value=a4
  Integrator : Integrator  InitialCondition=Tpo_init10
  Product : Product  Inputs=3
  Product1 : Product
  Tpo : Outport
  wires:
  Dtlm/1 -> Product1/2
  Integrator/1 -> Tpo/1, Add1/2  "Tpo"
  Product/1 -> Add/1
  Tpi/1 -> Add1/1
  Add1/1 -> Product/3
  Product1/1 -> Add/2
  Constant2/1 -> Product1/1
  Constant1/1 -> Product/1
  Add/1 -> Integrator/1  "dTpo/dt"
  Fp/1 -> Product/2

== system hx_model_alsop_PID/Subsystem/Subsystem2 ==
  Fc : Inport
  Tci : Inport  Port=2
  Dtlm : Inport  Port=3
  Add : Sum
  Add1 : Sum  Inputs=+-
  Constant1 : Constant  Value=a1
  Constant2 : Constant  Value=a2
  Integrator : Integrator  InitialCondition=Tco_init2
  Product : Product  Inputs=3
  Product1 : Product
  Tco : Outport
  wires:
  Fc/1 -> Product/2
  Add/1 -> Integrator/1  "dTco/dt"
  Constant1/1 -> Product/1
  Constant2/1 -> Product1/1
  Product1/1 -> Add/2
  Add1/1 -> Product/3
  Tci/1 -> Add1/1
  Product/1 -> Add/1
  Integrator/1 -> Add1/2, Tco/1  "Tco"
  Dtlm/1 -> Product1/2

== system hx_model_alsop_PID/Subsystem/Subsystem20 ==
  Fc : Inport
  Tci : Inport  Port=2
  Dtlm : Inport  Port=3
  Add : Sum
  Add1 : Sum  Inputs=+-
  Constant1 : Constant  Value=a1
  Constant2 : Constant  Value=a2
  Integrator : Integrator  InitialCondition=Tco_init11
  Product : Product  Inputs=3
  Product1 : Product
  Tco : Outport
  wires:
  Dtlm/1 -> Product1/2
  Integrator/1 -> Tco/1, Add1/2  "Tco"
  Product/1 -> Add/1
  Tci/1 -> Add1/1
  Add1/1 -> Product/3
  Product1/1 -> Add/2
  Constant2/1 -> Product1/1
  Constant1/1 -> Product/1
  Add/1 -> Integrator/1  "dTco/dt"
  Fc/1 -> Product/2

== system hx_model_alsop_PID/Subsystem/Subsystem21 ==
  Fp : Inport
  Tpi : Inport  Port=2
  Dtlm : Inport  Port=3
  Add : Sum  Inputs=+-
  Add1 : Sum  Inputs=+-
  Constant1 : Constant  Value=a3
  Constant2 : Constant  Value=a4
  Integrator : Integrator  InitialCondition=Tpo_init11
  Product : Product  Inputs=3
  Product1 : Product
  Tpo : Outport
  wires:
  Fp/1 -> Product/2
  Add/1 -> Integrator/1  "dTpo/dt"
  Constant1/1 -> Product/1
  Constant2/1 -> Product1/1
  Product1/1 -> Add/2
  Add1/1 -> Product/3
  Tpi/1 -> Add1/1
  Product/1 -> Add/1
  Integrator/1 -> Add1/2, Tpo/1  "Tpo"
  Dtlm/1 -> Product1/2

== system hx_model_alsop_PID/Subsystem/Subsystem22 ==
  Fc : Inport
  Tci : Inport  Port=2
  Dtlm : Inport  Port=3
  Add : Sum
  Add1 : Sum  Inputs=+-
  Constant1 : Constant  Value=a1
  Constant2 : Constant  Value=a2
  Integrator : Integrator  InitialCondition=Tco_init16
  Product : Product  Inputs=3
  Product1 : Product
  Tco : Outport
  wires:
  Fc/1 -> Product/2
  Add/1 -> Integrator/1  "dTco/dt"
  Constant1/1 -> Product/1
  Constant2/1 -> Product1/1
  Product1/1 -> Add/2
  Add1/1 -> Product/3
  Tci/1 -> Add1/1
  Product/1 -> Add/1
  Integrator/1 -> Add1/2, Tco/1  "Tco"
  Dtlm/1 -> Product1/2

== system hx_model_alsop_PID/Subsystem/Subsystem23 ==
  Fp : Inport
  Tpi : Inport  Port=2
  Dtlm : Inport  Port=3
  Add : Sum  Inputs=+-
  Add1 : Sum  Inputs=+-
  Constant1 : Constant  Value=a3
  Constant2 : Constant  Value=a4
  Integrator : Integrator  InitialCondition=Tpo_init16
  Product : Product  Inputs=3
  Product1 : Product
  Tpo : Outport
  wires:
  Dtlm/1 -> Product1/2
  Integrator/1 -> Tpo/1, Add1/2  "Tpo"
  Product/1 -> Add/1
  Tpi/1 -> Add1/1
  Add1/1 -> Product/3
  Product1/1 -> Add/2
  Constant2/1 -> Product1/1
  Constant1/1 -> Product/1
  Add/1 -> Integrator/1  "dTpo/dt"
  Fp/1 -> Product/2

== system hx_model_alsop_PID/Subsystem/Subsystem24 ==
  Fc : Inport
  Tci : Inport  Port=2
  Dtlm : Inport  Port=3
  Add : Sum
  Add1 : Sum  Inputs=+-
  Constant1 : Constant  Value=a1
  Constant2 : Constant  Value=a2
  Integrator : Integrator  InitialCondition=Tco_init17
  Product : Product  Inputs=3
  Product1 : Product
  Tco : Outport
  wires:
  Dtlm/1 -> Product1/2
  Integrator/1 -> Tco/1, Add1/2  "Tco"
  Product/1 -> Add/1
  Tci/1 -> Add1/1
  Add1/1 -> Product/3
  Product1/1 -> Add/2
  Constant2/1 -> Product1/1
  Constant1/1 -> Product/1
  Add/1 -> Integrator/1  "dTco/dt"
  Fc/1 -> Product/2

== system hx_model_alsop_PID/Subsystem/Subsystem25 ==
  Fp : Inport
  Tpi : Inport  Port=2
  Dtlm : Inport  Port=3
  Add : Sum  Inputs=+-
  Add1 : Sum  Inputs=+-
  Constant1 : Constant  Value=a3
  Constant2 : Constant  Value=a4
  Integrator : Integrator  InitialCondition=Tpo_init17
  Product : Product  Inputs=3
  Product1 : Product
  Tpo : Outport
  wires:
  Fp/1 -> Product/2
  Add/1 -> Integrator/1  "dTpo/dt"
  Constant1/1 -> Product/1
  Constant2/1 -> Product1/1
  Product1/1 -> Add/2
  Add1/1 -> Product/3
  Tpi/1 -> Add1/1
  Product/1 -> Add/1
  Integrator/1 -> Add1/2, Tpo/1  "Tpo"
  Dtlm/1 -> Product1/2

== system hx_model_alsop_PID/Subsystem/Subsystem26 ==
  Fc : Inport
  Tci : Inport  Port=2
  Dtlm : Inport  Port=3
  Add : Sum
  Add1 : Sum  Inputs=+-
  Constant1 : Constant  Value=a1
  Constant2 : Constant  Value=a2
  Integrator : Integrator  InitialCondition=Tco_init18
  Product : Product  Inputs=3
  Product1 : Product
  Tco : Outport
  wires:
  Fc/1 -> Product/2
  Add/1 -> Integrator/1  "dTco/dt"
  Constant1/1 -> Product/1
  Constant2/1 -> Product1/1
  Product1/1 -> Add/2
  Add1/1 -> Product/3
  Tci/1 -> Add1/1
  Product/1 -> Add/1
  Integrator/1 -> Add1/2, Tco/1  "Tco"
  Dtlm/1 -> Product1/2

== system hx_model_alsop_PID/Subsystem/Subsystem27 ==
  Fp : Inport
  Tpi : Inport  Port=2
  Dtlm : Inport  Port=3
  Add : Sum  Inputs=+-
  Add1 : Sum  Inputs=+-
  Constant1 : Constant  Value=a3
  Constant2 : Constant  Value=a4
  Integrator : Integrator  InitialCondition=Tpo_init18
  Product : Product  Inputs=3
  Product1 : Product
  Tpo : Outport
  wires:
  Dtlm/1 -> Product1/2
  Integrator/1 -> Tpo/1, Add1/2  "Tpo"
  Product/1 -> Add/1
  Tpi/1 -> Add1/1
  Add1/1 -> Product/3
  Product1/1 -> Add/2
  Constant2/1 -> Product1/1
  Constant1/1 -> Product/1
  Add/1 -> Integrator/1  "dTpo/dt"
  Fp/1 -> Product/2

== system hx_model_alsop_PID/Subsystem/Subsystem28 ==
  Fc : Inport
  Tci : Inport  Port=2
  Dtlm : Inport  Port=3
  Add : Sum
  Add1 : Sum  Inputs=+-
  Constant1 : Constant  Value=a1
  Constant2 : Constant  Value=a2
  Integrator : Integrator  InitialCondition=Tco_init19
  Product : Product  Inputs=3
  Product1 : Product
  Tco : Outport
  wires:
  Dtlm/1 -> Product1/2
  Integrator/1 -> Tco/1, Add1/2  "Tco"
  Product/1 -> Add/1
  Tci/1 -> Add1/1
  Add1/1 -> Product/3
  Product1/1 -> Add/2
  Constant2/1 -> Product1/1
  Constant1/1 -> Product/1
  Add/1 -> Integrator/1  "dTco/dt"
  Fc/1 -> Product/2

== system hx_model_alsop_PID/Subsystem/Subsystem29 ==
  Fp : Inport
  Tpi : Inport  Port=2
  Dtlm : Inport  Port=3
  Add : Sum  Inputs=+-
  Add1 : Sum  Inputs=+-
  Constant1 : Constant  Value=a3
  Constant2 : Constant  Value=a4
  Integrator : Integrator  InitialCondition=Tpo_init19
  Product : Product  Inputs=3
  Product1 : Product
  Tpo : Outport
  wires:
  Fp/1 -> Product/2
  Add/1 -> Integrator/1  "dTpo/dt"
  Constant1/1 -> Product/1
  Constant2/1 -> Product1/1
  Product1/1 -> Add/2
  Add1/1 -> Product/3
  Tpi/1 -> Add1/1
  Product/1 -> Add/1
  Integrator/1 -> Add1/2, Tpo/1  "Tpo"
  Dtlm/1 -> Product1/2

== system hx_model_alsop_PID/Subsystem/Subsystem3 ==
  Fp : Inport
  Tpi : Inport  Port=2
  Dtlm : Inport  Port=3
  Add : Sum  Inputs=+-
  Add1 : Sum  Inputs=+-
  Constant1 : Constant  Value=a3
  Constant2 : Constant  Value=a4
  Integrator : Integrator  InitialCondition=Tpo_init2
  Product : Product  Inputs=3
  Product1 : Product
  Tpo : Outport
  wires:
  Dtlm/1 -> Product1/2
  Integrator/1 -> Tpo/1, Add1/2  "Tpo"
  Product/1 -> Add/1
  Tpi/1 -> Add1/1
  Add1/1 -> Product/3
  Product1/1 -> Add/2
  Constant2/1 -> Product1/1
  Constant1/1 -> Product/1
  Add/1 -> Integrator/1  "dTpo/dt"
  Fp/1 -> Product/2

== system hx_model_alsop_PID/Subsystem/Subsystem30 ==
  Fc : Inport
  Tci : Inport  Port=2
  Dtlm : Inport  Port=3
  Add : Sum
  Add1 : Sum  Inputs=+-
  Constant1 : Constant  Value=a1
  Constant2 : Constant  Value=a2
  Integrator : Integrator  InitialCondition=Tco_init20
  Product : Product  Inputs=3
  Product1 : Product
  Tco : Outport
  wires:
  Fc/1 -> Product/2
  Add/1 -> Integrator/1  "dTco/dt"
  Constant1/1 -> Product/1
  Constant2/1 -> Product1/1
  Product1/1 -> Add/2
  Add1/1 -> Product/3
  Tci/1 -> Add1/1
  Product/1 -> Add/1
  Integrator/1 -> Add1/2, Tco/1  "Tco"
  Dtlm/1 -> Product1/2

== system hx_model_alsop_PID/Subsystem/Subsystem31 ==
  Fp : Inport
  Tpi : Inport  Port=2
  Dtlm : Inport  Port=3
  Add : Sum  Inputs=+-
  Add1 : Sum  Inputs=+-
  Constant1 : Constant  Value=a3
  Constant2 : Constant  Value=a4
  Integrator : Integrator  InitialCondition=Tpo_init20
  Product : Product  Inputs=3
  Product1 : Product
  Tpo : Outport
  wires:
  Dtlm/1 -> Product1/2
  Integrator/1 -> Tpo/1, Add1/2  "Tpo"
  Product/1 -> Add/1
  Tpi/1 -> Add1/1
  Add1/1 -> Product/3
  Product1/1 -> Add/2
  Constant2/1 -> Product1/1
  Constant1/1 -> Product/1
  Add/1 -> Integrator/1  "dTpo/dt"
  Fp/1 -> Product/2

== system hx_model_alsop_PID/Subsystem/Subsystem32 ==
  Fc : Inport
  Tci : Inport  Port=2
  Dtlm : Inport  Port=3
  Add : Sum
  Add1 : Sum  Inputs=+-
  Constant1 : Constant  Value=a1
  Constant2 : Constant  Value=a2
  Integrator : Integrator  InitialCondition=Tco_init12
  Product : Product  Inputs=3
  Product1 : Product
  Tco : Outport
  wires:
  Fc/1 -> Product/2
  Add/1 -> Integrator/1  "dTco/dt"
  Constant1/1 -> Product/1
  Constant2/1 -> Product1/1
  Product1/1 -> Add/2
  Add1/1 -> Product/3
  Tci/1 -> Add1/1
  Product/1 -> Add/1
  Integrator/1 -> Add1/2, Tco/1  "Tco"
  Dtlm/1 -> Product1/2

== system hx_model_alsop_PID/Subsystem/Subsystem33 ==
  Fp : Inport
  Tpi : Inport  Port=2
  Dtlm : Inport  Port=3
  Add : Sum  Inputs=+-
  Add1 : Sum  Inputs=+-
  Constant1 : Constant  Value=a3
  Constant2 : Constant  Value=a4
  Integrator : Integrator  InitialCondition=Tpo_init12
  Product : Product  Inputs=3
  Product1 : Product
  Tpo : Outport
  wires:
  Dtlm/1 -> Product1/2
  Integrator/1 -> Tpo/1, Add1/2  "Tpo"
  Product/1 -> Add/1
  Tpi/1 -> Add1/1
  Add1/1 -> Product/3
  Product1/1 -> Add/2
  Constant2/1 -> Product1/1
  Constant1/1 -> Product/1
  Add/1 -> Integrator/1  "dTpo/dt"
  Fp/1 -> Product/2

== system hx_model_alsop_PID/Subsystem/Subsystem34 ==
  Fc : Inport
  Tci : Inport  Port=2
  Dtlm : Inport  Port=3
  Add : Sum
  Add1 : Sum  Inputs=+-
  Constant1 : Constant  Value=a1
  Constant2 : Constant  Value=a2
  Integrator : Integrator  InitialCondition=Tco_init13
  Product : Product  Inputs=3
  Product1 : Product
  Tco : Outport
  wires:
  Dtlm/1 -> Product1/2
  Integrator/1 -> Tco/1, Add1/2  "Tco"
  Product/1 -> Add/1
  Tci/1 -> Add1/1
  Add1/1 -> Product/3
  Product1/1 -> Add/2
  Constant2/1 -> Product1/1
  Constant1/1 -> Product/1
  Add/1 -> Integrator/1  "dTco/dt"
  Fc/1 -> Product/2

== system hx_model_alsop_PID/Subsystem/Subsystem35 ==
  Fp : Inport
  Tpi : Inport  Port=2
  Dtlm : Inport  Port=3
  Add : Sum  Inputs=+-
  Add1 : Sum  Inputs=+-
  Constant1 : Constant  Value=a3
  Constant2 : Constant  Value=a4
  Integrator : Integrator  InitialCondition=Tpo_init13
  Product : Product  Inputs=3
  Product1 : Product
  Tpo : Outport
  wires:
  Fp/1 -> Product/2
  Add/1 -> Integrator/1  "dTpo/dt"
  Constant1/1 -> Product/1
  Constant2/1 -> Product1/1
  Product1/1 -> Add/2
  Add1/1 -> Product/3
  Tpi/1 -> Add1/1
  Product/1 -> Add/1
  Integrator/1 -> Add1/2, Tpo/1  "Tpo"
  Dtlm/1 -> Product1/2

== system hx_model_alsop_PID/Subsystem/Subsystem36 ==
  Fc : Inport
  Tci : Inport  Port=2
  Dtlm : Inport  Port=3
  Add : Sum
  Add1 : Sum  Inputs=+-
  Constant1 : Constant  Value=a1
  Constant2 : Constant  Value=a2
  Integrator : Integrator  InitialCondition=Tco_init14
  Product : Product  Inputs=3
  Product1 : Product
  Tco : Outport
  wires:
  Fc/1 -> Product/2
  Add/1 -> Integrator/1  "dTco/dt"
  Constant1/1 -> Product/1
  Constant2/1 -> Product1/1
  Product1/1 -> Add/2
  Add1/1 -> Product/3
  Tci/1 -> Add1/1
  Product/1 -> Add/1
  Integrator/1 -> Add1/2, Tco/1  "Tco"
  Dtlm/1 -> Product1/2

== system hx_model_alsop_PID/Subsystem/Subsystem37 ==
  Fp : Inport
  Tpi : Inport  Port=2
  Dtlm : Inport  Port=3
  Add : Sum  Inputs=+-
  Add1 : Sum  Inputs=+-
  Constant1 : Constant  Value=a3
  Constant2 : Constant  Value=a4
  Integrator : Integrator  InitialCondition=Tpo_init14
  Product : Product  Inputs=3
  Product1 : Product
  Tpo : Outport
  wires:
  Dtlm/1 -> Product1/2
  Integrator/1 -> Tpo/1, Add1/2  "Tpo"
  Product/1 -> Add/1
  Tpi/1 -> Add1/1
  Add1/1 -> Product/3
  Product1/1 -> Add/2
  Constant2/1 -> Product1/1
  Constant1/1 -> Product/1
  Add/1 -> Integrator/1  "dTpo/dt"
  Fp/1 -> Product/2

== system hx_model_alsop_PID/Subsystem/Subsystem38 ==
  Fc : Inport
  Tci : Inport  Port=2
  Dtlm : Inport  Port=3
  Add : Sum
  Add1 : Sum  Inputs=+-
  Constant1 : Constant  Value=a1
  Constant2 : Constant  Value=a2
  Integrator : Integrator  InitialCondition=Tco_init15
  Product : Product  Inputs=3
  Product1 : Product
  Tco : Outport
  wires:
  Dtlm/1 -> Product1/2
  Integrator/1 -> Tco/1, Add1/2  "Tco"
  Product/1 -> Add/1
  Tci/1 -> Add1/1
  Add1/1 -> Product/3
  Product1/1 -> Add/2
  Constant2/1 -> Product1/1
  Constant1/1 -> Product/1
  Add/1 -> Integrator/1  "dTco/dt"
  Fc/1 -> Product/2

== system hx_model_alsop_PID/Subsystem/Subsystem39 ==
  Fp : Inport
  Tpi : Inport  Port=2
  Dtlm : Inport  Port=3
  Add : Sum  Inputs=+-
  Add1 : Sum  Inputs=+-
  Constant1 : Constant  Value=a3
  Constant2 : Constant  Value=a4
  Integrator : Integrator  InitialCondition=Tpo_init15
  Product : Product  Inputs=3
  Product1 : Product
  Tpo : Outport
  wires:
  Fp/1 -> Product/2
  Add/1 -> Integrator/1  "dTpo/dt"
  Constant1/1 -> Product/1
  Constant2/1 -> Product1/1
  Product1/1 -> Add/2
  Add1/1 -> Product/3
  Tpi/1 -> Add1/1
  Product/1 -> Add/1
  Integrator/1 -> Add1/2, Tpo/1  "Tpo"
  Dtlm/1 -> Product1/2

== system hx_model_alsop_PID/Subsystem/Subsystem4 ==
  Fc : Inport
  Tci : Inport  Port=2
  Dtlm : Inport  Port=3
  Add : Sum
  Add1 : Sum  Inputs=+-
  Constant1 : Constant  Value=a1
  Constant2 : Constant  Value=a2
  Integrator : Integrator  InitialCondition=Tco_init3
  Product : Product  Inputs=3
  Product1 : Product
  Tco : Outport
  wires:
  Dtlm/1 -> Product1/2
  Integrator/1 -> Tco/1, Add1/2  "Tco"
  Product/1 -> Add/1
  Tci/1 -> Add1/1
  Add1/1 -> Product/3
  Product1/1 -> Add/2
  Constant2/1 -> Product1/1
  Constant1/1 -> Product/1
  Add/1 -> Integrator/1  "dTco/dt"
  Fc/1 -> Product/2

== system hx_model_alsop_PID/Subsystem/Subsystem5 ==
  Fp : Inport
  Tpi : Inport  Port=2
  Dtlm : Inport  Port=3
  Add : Sum  Inputs=+-
  Add1 : Sum  Inputs=+-
  Constant1 : Constant  Value=a3
  Constant2 : Constant  Value=a4
  Integrator : Integrator  InitialCondition=Tpo_init3
  Product : Product  Inputs=3
  Product1 : Product
  Tpo : Outport
  wires:
  Fp/1 -> Product/2
  Add/1 -> Integrator/1  "dTpo/dt"
  Constant1/1 -> Product/1
  Constant2/1 -> Product1/1
  Product1/1 -> Add/2
  Add1/1 -> Product/3
  Tpi/1 -> Add1/1
  Product/1 -> Add/1
  Integrator/1 -> Add1/2, Tpo/1  "Tpo"
  Dtlm/1 -> Product1/2

== system hx_model_alsop_PID/Subsystem/Subsystem6 ==
  Fc : Inport
  Tci : Inport  Port=2
  Dtlm : Inport  Port=3
  Add : Sum
  Add1 : Sum  Inputs=+-
  Constant1 : Constant  Value=a1
  Constant2 : Constant  Value=a2
  Integrator : Integrator  InitialCondition=Tco_init4
  Product : Product  Inputs=3
  Product1 : Product
  Tco : Outport
  wires:
  Fc/1 -> Product/2
  Add/1 -> Integrator/1  "dTco/dt"
  Constant1/1 -> Product/1
  Constant2/1 -> Product1/1
  Product1/1 -> Add/2
  Add1/1 -> Product/3
  Tci/1 -> Add1/1
  Product/1 -> Add/1
  Integrator/1 -> Add1/2, Tco/1  "Tco"
  Dtlm/1 -> Product1/2

== system hx_model_alsop_PID/Subsystem/Subsystem7 ==
  Fp : Inport
  Tpi : Inport  Port=2
  Dtlm : Inport  Port=3
  Add : Sum  Inputs=+-
  Add1 : Sum  Inputs=+-
  Constant1 : Constant  Value=a3
  Constant2 : Constant  Value=a4
  Integrator : Integrator  InitialCondition=Tpo_init4
  Product : Product  Inputs=3
  Product1 : Product
  Tpo : Outport
  wires:
  Dtlm/1 -> Product1/2
  Integrator/1 -> Tpo/1, Add1/2  "Tpo"
  Product/1 -> Add/1
  Tpi/1 -> Add1/1
  Add1/1 -> Product/3
  Product1/1 -> Add/2
  Constant2/1 -> Product1/1
  Constant1/1 -> Product/1
  Add/1 -> Integrator/1  "dTpo/dt"
  Fp/1 -> Product/2

== system hx_model_alsop_PID/Subsystem/Subsystem8 ==
  Fc : Inport
  Tci : Inport  Port=2
  Dtlm : Inport  Port=3
  Add : Sum
  Add1 : Sum  Inputs=+-
  Constant1 : Constant  Value=a1
  Constant2 : Constant  Value=a2
  Integrator : Integrator  InitialCondition=Tco_init5
  Product : Product  Inputs=3
  Product1 : Product
  Tco : Outport
  wires:
  Dtlm/1 -> Product1/2
  Integrator/1 -> Tco/1, Add1/2  "Tco"
  Product/1 -> Add/1
  Tci/1 -> Add1/1
  Add1/1 -> Product/3
  Product1/1 -> Add/2
  Constant2/1 -> Product1/1
  Constant1/1 -> Product/1
  Add/1 -> Integrator/1  "dTco/dt"
  Fc/1 -> Product/2

== system hx_model_alsop_PID/Subsystem/Subsystem9 ==
  Fp : Inport
  Tpi : Inport  Port=2
  Dtlm : Inport  Port=3
  Add : Sum  Inputs=+-
  Add1 : Sum  Inputs=+-
  Constant1 : Constant  Value=a3
  Constant2 : Constant  Value=a4
  Integrator : Integrator  InitialCondition=Tpo_init5
  Product : Product  Inputs=3
  Product1 : Product
  Tpo : Outport
  wires:
  Fp/1 -> Product/2
  Add/1 -> Integrator/1  "dTpo/dt"
  Constant1/1 -> Product/1
  Constant2/1 -> Product1/1
  Product1/1 -> Add/2
  Add1/1 -> Product/3
  Tpi/1 -> Add1/1
  Product/1 -> Add/1
  Integrator/1 -> Add1/2, Tpo/1  "Tpo"
  Dtlm/1 -> Product1/2

== matlab function hx_model_alsop_PID/Subsystem/MATLAB Function1 ==
  data: Tpi input; DeltaT_LM output; Tco input; Tpo input; Tci input
function DeltaT_LM = fcn(Tpi,Tco,Tpo,Tci)
    Delta_T1 = Tpi-Tco;
    Delta_T2 = Tpo-Tci;
    if Delta_T1~=Delta_T2
        DeltaT_LM = (Delta_T1-Delta_T2)/log(Delta_T1/Delta_T2);
    else
        DeltaT_LM = Delta_T1;
    end
end

== matlab function hx_model_alsop_PID/Subsystem/MATLAB Function ==
  data: Tpi input; DeltaT_LM output; Tco input; Tpo input; Tci input
function DeltaT_LM = fcn(Tpi,Tco,Tpo,Tci)
    Delta_T1 = Tpi-Tco;
    Delta_T2 = Tpo-Tci;
    if Delta_T1~=Delta_T2
        DeltaT_LM = (Delta_T1-Delta_T2)/log(Delta_T1/Delta_T2);
    else
        DeltaT_LM = Delta_T1;
    end
end

== matlab function hx_model_alsop_PID/Subsystem/MATLAB Function2 ==
  data: Tpi input; DeltaT_LM output; Tco input; Tpo input; Tci input
function DeltaT_LM = fcn(Tpi,Tco,Tpo,Tci)
    Delta_T1 = Tpi-Tco;
    Delta_T2 = Tpo-Tci;
    if Delta_T1~=Delta_T2
        DeltaT_LM = (Delta_T1-Delta_T2)/log(Delta_T1/Delta_T2);
    else
        DeltaT_LM = Delta_T1;
    end
end

== matlab function hx_model_alsop_PID/Subsystem/MATLAB Function3 ==
  data: Tpi input; DeltaT_LM output; Tco input; Tpo input; Tci input
function DeltaT_LM = fcn(Tpi,Tco,Tpo,Tci)
    Delta_T1 = Tpi-Tco;
    Delta_T2 = Tpo-Tci;
    if Delta_T1~=Delta_T2
        DeltaT_LM = (Delta_T1-Delta_T2)/log(Delta_T1/Delta_T2);
    else
        DeltaT_LM = Delta_T1;
    end
end
